simulink model "modele_bo"  (R2025b)
settings: Solver=VariableStepAuto  StartTime=0.0  StopTime=10.0  RelTol=1e-3
values from neighbouring files (symbols this model uses):
  d1_nom = 3.12    [variables.m]
  d2 = 3.73    [variables.m]
  k = k + nzb    [kron.m]    (also in variables.m = 400)
  km = 2.96    [variables.m]
  ky = 280    [variables.m]
  m1 = 2.29    [variables.m]
  m2 = 2.044    [variables.m]
settings Model: Creator=flo  LastModifiedBy=flo

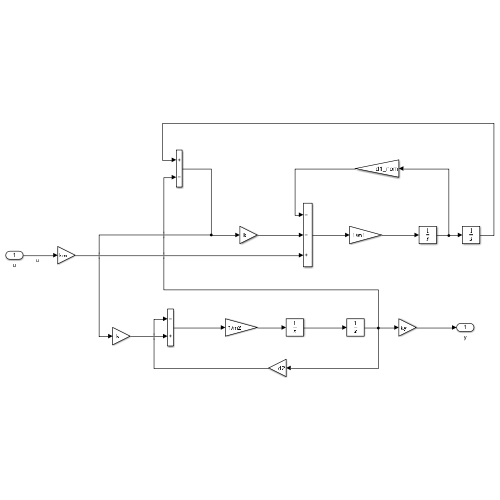
[thumbnail: Simulink's stored preview of the top-level diagram]
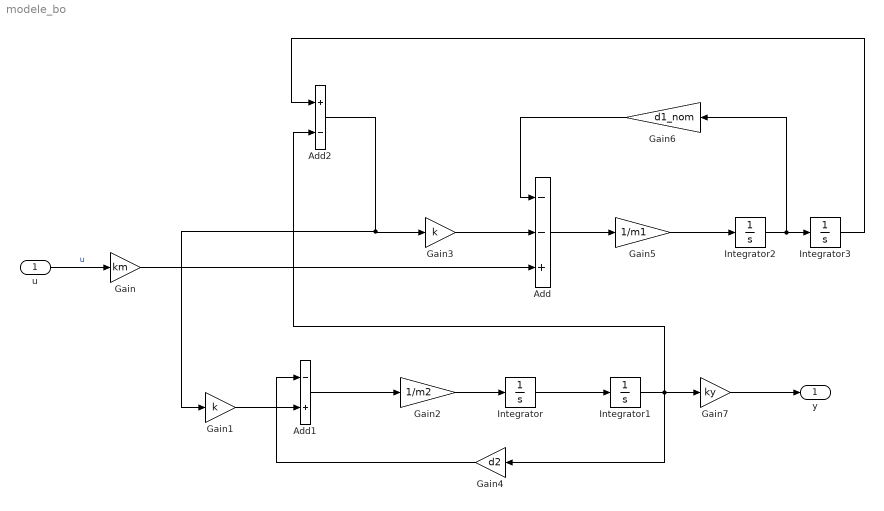
== system modele_bo ==
  u : Inport
  Add : Sum  Inputs=--+
  Add1 : Sum  Inputs=-+
  Add2 : Sum  Inputs=+-
  Gain : Gain  Gain=km
  Gain1 : Gain  Gain=k
  Gain2 : Gain  Gain=1/m2
  Gain3 : Gain  Gain=k
  Gain4 : Gain  Gain=d2
  Gain5 : Gain  Gain=1/m1
  Gain6 : Gain  Gain=d1_nom
  Gain7 : Gain  Gain=ky
  Integrator{,1..3} (4 alike) : Integrator
  y : Outport
  wires:
  Gain/1 -> Add/3
  u/1 -> Gain/1  "u"
  Gain1/1 -> Add1/2
  Add1/1 -> Gain2/1
  Gain3/1 -> Add/2
  Gain2/1 -> Integrator/1
  Integrator/1 -> Integrator1/1
  Integrator1/1 -> Gain7/1, Gain4/1, Add2/2
  Gain4/1 -> Add1/1
  Add2/1 -> Gain1/1, Gain3/1
  Add/1 -> Gain5/1
  Gain5/1 -> Integrator2/1
  Integrator2/1 -> Gain6/1, Integrator3/1
  Gain6/1 -> Add/1
  Integrator3/1 -> Add2/1
  Gain7/1 -> y/1
